simulink model "Control_schemes_2019b"  (R2021a)
settings: Solver=VariableStepAuto  StartTime=0.0  StopTime=10  RelTol=1e-3
values from neighbouring files (symbols this model uses):
  K_lqr = lqr(sysestc,Q,R)    [Controller.m]    (also in LQR_Controller.m)
undefined symbols (not defined in the file or in its folder): sigbuilder_block, v_a_max
libraries: simulink_extras x7, cstblocks x5
settings Model: Creator=AleFire  LastModifiedBy=arco
settings SolverCC: AlgebraicLoopSolver=TrustRegion
settings DebuggingCC: UnconnectedInputMsg=none  UnconnectedOutputMsg=none  UnconnectedLineMsg=none
settings ModelReferenceCC: EnableRefExpFcnMdlSchedulingChecks=off
settings RTWCC: Description=Generic Real-Time Target

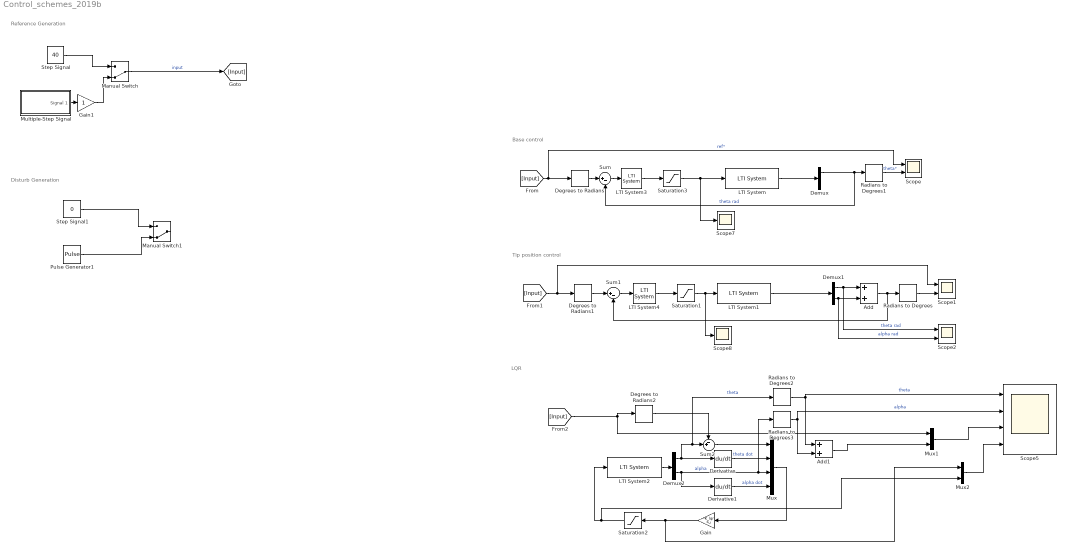
== system Control_schemes_2019b ==
  note: LQR
  note: Tip position control
  note: Base control
  note: Disturb Generation
  note: Reference Generation
  Add : Sum
  Add1 : Sum
  Degrees to Radians : simulink_extras/Transformations/Degrees to Radians
  Degrees to Radians1 : simulink_extras/Transformations/Degrees to Radians
  Degrees to Radians2 : simulink_extras/Transformations/Degrees to Radians
  Demux : Demux  Outputs=2
  Demux1 : Demux  Outputs=2
  Demux2 : Demux  Outputs=2
  Derivative : Derivative
  Derivative1 : Derivative
  Gain : Gain  Gain=-K_lqr  Multiplication=Matrix(K*u)
  Gain1 : Gain
  LTI System : cstblocks/LTI System  sys=sysestc  IC=[]
  LTI System1 : cstblocks/LTI System  sys=sysestc  IC=[]
  LTI System2 : cstblocks/LTI System  sys=sysestc  IC=[]
  LTI System3 : cstblocks/LTI System  sys=C_comp  IC=[]
  LTI System4 : cstblocks/LTI System  sys=C_comp  IC=[]
  Manual Switch : ManualSwitch  CurrentSetting=0
  Manual Switch1 : ManualSwitch  CurrentSetting=0
  Multiple-Step Signal : Subsystem  Tag=STV Subsys  LoadFcn=sigbuilder_block('load');  StartFcn=sigbuilder_block('start');  StopFcn=sigbuilder_block('stop');  ClipboardFcn=sigbuilder_block('clipboard');  mask(Sigbuilder block){tuvar=[0:10]}
      mask help: Simulink:masks:SigbuilderBlock_MD
      mask init:
      | if ~strcmp(get_param(bdroot(gcbh),'SimulationStatus'),'stopped') tuvar = sigbuilder_block('maskInit'); end
      settings: CopyFcn=sigbuilder_block('copy');  DeleteFcn=sigbuilder_block('delete');  ModelCloseFcn=sigbuilder_block('modelClose');  PreSaveFcn=sigbuilder_block('preSave');  PauseFcn=sigbuilder_block('pause');  ContinueFcn=sigbuilder_block('continue');  NameChangeFcn=sigbuilder_block('namechange');  OpenFcn=sigbuilder_block('open',[-116 1261 550 400 ]);  CloseFcn=sigbuilder_block('close');
      mask Display: plot(0, 0, 100, 100,[2, 2, 32, 32, 2], [68, 8, 8, 68, 68],[32, 2], [38, 38], [32, 19, 2],[53, 60, 44], [32, 17, 17, 2],[16, 16, 31, 31]);txt = getActiveGroup(gcbh);text(2, 100, txt,'verticalAlignment', 'top');
  Mux : Mux
  Mux1 : Mux  Inputs=2
  Mux2 : Mux  Inputs=2
  Pulse Generator1 : DiscretePulseGenerator  PulseType=Time based  Amplitude=.2  Period=1.5  PulseWidth=5
  Radians to Degrees{,1..3} (4 alike) : simulink_extras/Transformations/Radians to Degrees
  Saturation1 : Saturate  UpperLimit=v_a_max  LowerLimit=-v_a_max
  Saturation2 : Saturate  UpperLimit=v_a_max  LowerLimit=-v_a_max
  Saturation3 : Saturate  UpperLimit=v_a_max  LowerLimit=-v_a_max
  Scope : Scope  NumInputPorts=2
  Scope1 : Scope  NumInputPorts=2
  Scope2 : Scope  NumInputPorts=2
  Scope5 : Scope  NumInputPorts=4
  Scope7 : Scope
  Scope8 : Scope
  Step Signal : Constant  Value=40
  Step Signal1 : Constant  Value=0
  Sum : Sum  Inputs=|+-
  Sum1 : Sum  Inputs=|+-
  Sum2 : Sum  Inputs=-+|
  wires:
  [Input] -> Degrees to Radians/1, Scope/1  "ref°"
  Degrees to Radians/1 -> Sum/1
  Demux/1 -> Radians to Degrees1/1, Sum/2  "theta rad"
  LTI System/1 -> Demux/1
  Radians to Degrees1/1 -> Scope/2  "theta°"
  Radians to Degrees/1 -> Scope1/2
  Add/1 -> Radians to Degrees/1, Sum1/2
  LTI System1/1 -> Demux1/1
  Degrees to Radians1/1 -> Sum1/1
  [Input] -> Degrees to Radians1/1, Scope1/1
  Demux1/1 -> Scope2/1, Add/1  "theta rad"
  Demux1/2 -> Scope2/2, Add/2  "alpha rad"
  Degrees to Radians2/1 -> Sum2/1
  LTI System2/1 -> Demux2/1
  Demux2/1 -> Radians to Degrees2/1, Sum2/2, Derivative/1  "theta"
  Derivative/1 -> Mux/2  "theta dot"
  Mux/1 -> Gain/1
  Demux2/2 -> Derivative1/1, Radians to Degrees3/1, Mux/3  "alpha"
  Derivative1/1 -> Mux/4  "alpha dot"
  Sum2/1 -> Mux/1
  Radians to Degrees2/1 -> Add1/1, Scope5/1  "theta"
  Radians to Degrees3/1 -> Scope5/2, Add1/2  "alpha"
  Add1/1 -> Mux1/2
  [Input] -> Mux1/1, Degrees to Radians2/1
  Sum1/1 -> LTI System4/1
  Sum/1 -> LTI System3/1
  LTI System3/1 -> Saturation3/1
  Saturation3/1 -> Scope7/1, LTI System/1
  Saturation1/1 -> Scope8/1, LTI System1/1
  LTI System4/1 -> Saturation1/1
  Saturation2/1 -> Mux2/2, LTI System2/1
  Pulse Generator1/1 -> Manual Switch1/2
  Step Signal1/1 -> Manual Switch1/1
  Step Signal/1 -> Manual Switch/1
  Gain1/1 -> Manual Switch/2
  Manual Switch/1 -> [Input]  "input"
  Mux1/1 -> Scope5/3
  Gain/1 -> Mux2/1, Saturation2/1
  Multiple-Step Signal/1(Signal 1) -> Gain1/1
  Mux2/1 -> Scope5/4

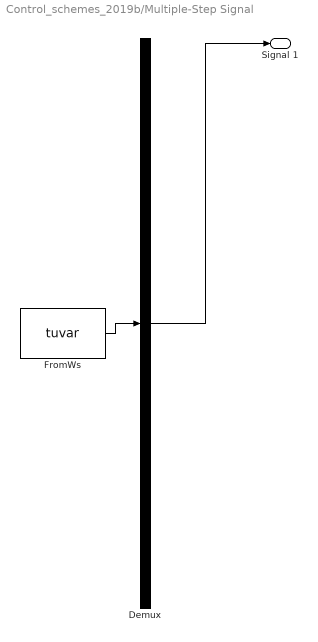
== system Control_schemes_2019b/Multiple-Step Signal ==
  Demux : Demux  Tag=STV Demux  Outputs=1
      settings: DisplayOption=none
  FromWs : FromWorkspace  Tag=STV FromWs  VariableName=tuvar
      SigBuilderData=|
      | common.afterFinalStr = 'Extrapolate'
      | common.sampleTime = 0
      | dataSet.timeRange = [0 10]
      | dataSet.name = 'Group 1'
      | sbobj.Groups.Name = 'Group 1'
      | sbobj.Groups.Signals.Name = 'Signal 1'
      | sbobj.Groups.Signals.XData = [0 1 1 3 3 5 5 7 7 8.5 8.5 10]
      | sbobj.Groups.Signals.YData = [0.005 0.005 40 40 15 15 -30 -30 0 0 23 23]
  Signal 1 : Outport  Tag=STV Outport
  wires:
  Demux/1 -> Signal 1/1
  FromWs/1 -> Demux/1
